simulink model "PID_perturbaciones"  (R2015a)
settings: Solver=ode45  StartTime=0.0  StopTime=1.5  RelTol=1e-3
values from neighbouring files (symbols this model uses):
  Ki1 = 0    [Inicio.m]
  Ki2 = 0    [Inicio.m]
  Ki3 = 0    [Inicio.m]
  Ki4 = 0    [Inicio.m]
  Kp1 = 200    [Inicio.m]
  Kp2 = 200    [Inicio.m]
  Kp3 = 200    [Inicio.m]
  Kp4 = 200    [Inicio.m]
  Kv1 = 50    [Inicio.m]
  Kv2 = 50    [Inicio.m]
  Kv3 = 50    [Inicio.m]
  Kv4 = 50    [Inicio.m]
  Tem = 0.0001    [Inicio.m]
settings Model: CovHtmlReporting=off  Creator=ANDRES Y MARCELA  LastModifiedBy=Shadow
settings DataIOCC: SignalLoggingSaveFormat=ModelDataLogs
settings OptimizationCC: ExpressionDepthLimit=2147483647
settings DebuggingCC: UnderspecifiedInitializationDetection=Classic  MergeDetectMultiDrivingBlocksExec=none  SolverPrmCheckMsg=warning  FcnCallInpInsideContextMsg=EnableAllAsWarning  StateNameClashWarn=warning
settings GRTTargetCC: CombineOutputUpdateFcns=off  GRTInterface=on

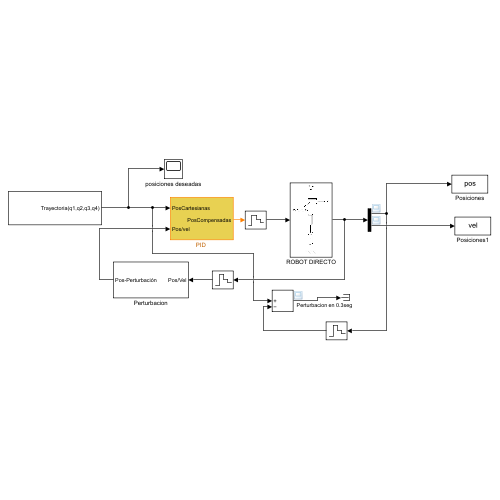
[thumbnail: Simulink's stored preview of the top-level diagram]
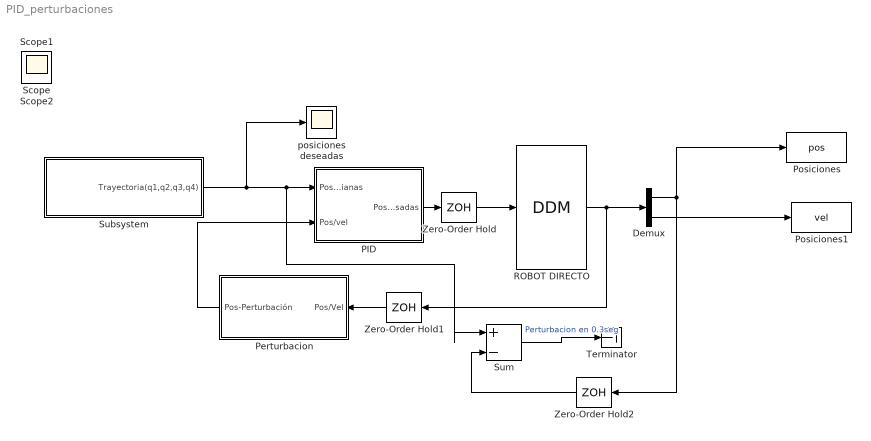
== system PID_perturbaciones ==
  Demux : Demux  Outputs=2
  "PID " : Subsystem
  Perturbacion : Subsystem
  Posiciones : ToWorkspace  VariableName=pos  SampleTime=-1
  Posiciones1 : ToWorkspace  VariableName=vel  SampleTime=-1
  ROBOT DIRECTO : S-Function  FunctionName=DDM  Parameters=QI  SFunctionDeploymentMode=off  EnableBusSupport=off
      mask Display: image(imread('robot.jpg'))
  Subsystem : Subsystem
  Sum : Sum  Inputs=|+-
  Terminator : Terminator
  Zero-Order Hold : ZeroOrderHold  SampleTime=Tem
  Zero-Order Hold1 : ZeroOrderHold  SampleTime=Tem
  Zero-Order Hold2 : ZeroOrderHold  SampleTime=Tem
  posiciones deseadas : Scope
      settings: TimeRange=auto  LimitDataPoints=on  MaxDataPoints=5000  SaveToWorkspace=off  SaveName=ScopeData2  YMin=0.7125  YMax=1.5875  SampleTime=-1
  Scope : Scope
      settings: TimeRange=auto  MaxDataPoints=5000  SaveToWorkspace=off  YMin=-0.18771  YMax=1.68049  SampleTime=-1
  Scope1 : Scope
      settings: TimeRange=auto  MaxDataPoints=5000  SaveToWorkspace=off  SaveName=ScopeData2  YMin=-0.0546  YMax=0.15744  SampleTime=-1
  Scope2 : Scope
      settings: TimeRange=auto  MaxDataPoints=5000  SaveToWorkspace=off  SaveName=ScopeData3  YMin=-1.04714  YMax=6.21183  SampleTime=-1
  wires:
  ROBOT DIRECTO/1 -> Zero-Order Hold1/1, Demux/1
  Demux/1 -> Zero-Order Hold2/1, Posiciones/1
  Demux/2 -> Posiciones1/1
  "PID "/1(PosCompensadas) -> Zero-Order Hold/1
  Zero-Order Hold/1 -> ROBOT DIRECTO/1
  Zero-Order Hold1/1 -> Perturbacion/1(Pos/Vel)
  Perturbacion/1(Pos-Perturbación) -> "PID "/2(Pos/vel)
  Zero-Order Hold2/1 -> Sum/2
  Subsystem/1(Trayectoria(q1,q2,q3,q4)) -> posiciones deseadas/1, Sum/1, "PID "/1(PosCartesianas)
  Sum/1 -> Terminator/1  "Perturbacion en 0.3seg"

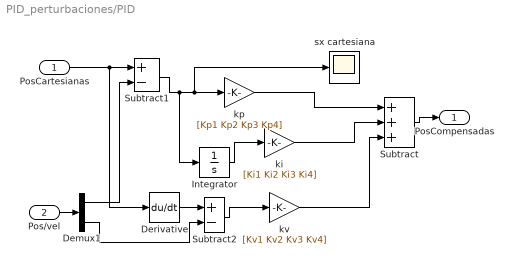
== system PID_perturbaciones/PID  ==
  PosCartesianas : Inport
  Pos/vel : Inport  Port=2
  Demux1 : Demux  Outputs=2
  Derivative : Derivative
  Integrator : Integrator
  Subtract : Sum  Inputs=+++
  Subtract1 : Sum  Inputs=+-
  Subtract2 : Sum  Inputs=+-
  ki : Gain  Gain=[Ki1 Ki2 Ki3 Ki4]
  kp : Gain  Gain=[Kp1 Kp2 Kp3 Kp4]
  kv : Gain  Gain=[Kv1 Kv2 Kv3 Kv4]
  sx cartesiana : Scope
      settings: TimeRange=auto  LimitDataPoints=on  MaxDataPoints=5000  SaveToWorkspace=off  YMin=-0.24887  YMax=0.22424  SampleTime=-1
  PosCompensadas : Outport
  wires:
  Subtract1/1 -> Integrator/1, kp/1, sx cartesiana/1
  Derivative/1 -> Subtract2/1
  Subtract2/1 -> kv/1
  kp/1 -> Subtract/1
  Integrator/1 -> ki/1
  Pos/vel/1 -> Demux1/1
  PosCartesianas/1 -> Derivative/1, Subtract1/1
  Subtract/1 -> PosCompensadas/1
  Demux1/1 -> Subtract1/2
  Demux1/2 -> Subtract2/2
  ki/1 -> Subtract/2
  kv/1 -> Subtract/3

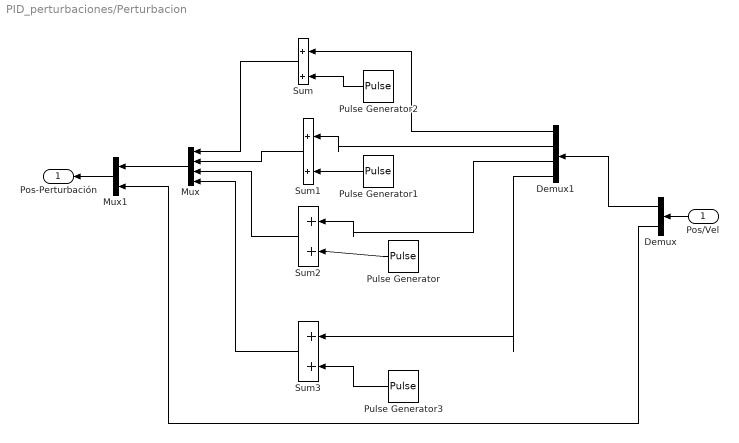
== system PID_perturbaciones/Perturbacion ==
  Pos/Vel : Inport
  Demux : Demux  Outputs=2
  Demux1 : Demux
  Mux : Mux
  Mux1 : Mux  Inputs=2
  Pulse Generator{,1..3} (4 alike) : DiscretePulseGenerator  PulseType=Time based  Amplitude=0.5  Period=10  PulseWidth=0.1  PhaseDelay=0.3
  Sum{,1..3} (4 alike) : Sum  Inputs=|++
  Pos-Perturbación : Outport
  wires:
  Demux/1 -> Demux1/1
  Demux1/1 -> Sum/1
  Pulse Generator2/1 -> Sum/2
  Pulse Generator1/1 -> Sum1/2
  Demux1/2 -> Sum1/1
  Demux1/3 -> Sum2/1
  Pulse Generator/1 -> Sum2/2
  Sum/1 -> Mux/1
  Sum1/1 -> Mux/2
  Sum2/1 -> Mux/3
  Mux/1 -> Mux1/1
  Demux/2 -> Mux1/2
  Mux1/1 -> Pos-Perturbación/1
  Pos/Vel/1 -> Demux/1
  Sum3/1 -> Mux/4
  Demux1/4 -> Sum3/1
  Pulse Generator3/1 -> Sum3/2

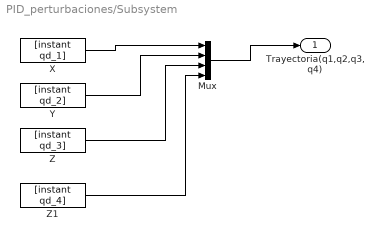
== system PID_perturbaciones/Subsystem ==
  Mux : Mux
  X : FromWorkspace  VariableName=[instant qd_1]  SampleTime=Tem
  Y : FromWorkspace  VariableName=[instant qd_2]  SampleTime=Tem
  Z : FromWorkspace  VariableName=[instant qd_3]  SampleTime=Tem
  Z1 : FromWorkspace  VariableName=[instant qd_4]  SampleTime=Tem
  Trayectoria(q1,q2,q3,q4) : Outport
  wires:
  Y/1 -> Mux/2
  Z/1 -> Mux/3
  X/1 -> Mux/1
  Mux/1 -> Trayectoria(q1,q2,q3,q4)/1
  Z1/1 -> Mux/4
